simulink model "AllinOne_2014a"  (R2014a)
settings: Solver=ode3  SolverMode=SingleTasking  StartTime=0.0  StopTime=Inf  RelTol=1e-3
StopFcn:
  | CoffeeMachineIOSupport('closefig');
settings Model: DataDictionary=Struct.sldd  NumberOfSteps=100  ParamWorkspaceSource=ReferencedWorkspace  Creator=89YY  LastModifiedBy=zhiping
settings OptimizationCC: InlineParams=on  UseFloatMulNetSlope=on  InlineInvariantSignals=on  PassReuseOutputArgsAs=Individual arguments  ZeroExternalMemoryAtStartup=off  ZeroInternalMemoryAtStartup=off  NoFixptDivByZeroProtection=on  EfficientFloat2IntCast=on  OptimizeModelRefInitCode=on  LifeSpan=1
settings DebuggingCC: SaveWithParameterizedLinksMsg=none  UnderspecifiedInitializationDetection=Classic  SolverPrmCheckMsg=none  FrameProcessingCompatibilityMsg=error
settings HardwareCC: ProdBitPerPointer=64  ProdLargestAtomicFloat=Float  ProdIntDivRoundTo=Zero  ProdEndianess=LittleEndian  ProdHWDeviceType=Specified  TargetBitPerPointer=64  TargetLongLongMode=on  TargetIntDivRoundTo=Zero  TargetEndianess=LittleEndian  TargetWordSize=64  TargetHWDeviceType=MATLAB Host  ProdEqTarget=off
settings RTWCC: SystemTargetFile=ert.tlc  TemplateMakefile=ert_default_tmf  Description=Embedded Coder  GenerateReport=on  IncludeHyperlinkInReport=on  LaunchReport=on  GenerateTraceInfo=on  GenerateTraceReport=on  GenerateTraceReportSl=on  GenerateTraceReportSf=on  GenerateTraceReportEml=on  GenerateCodeMetricsReport=on
settings CodeAppCC: ForceParamTrailComments=on  IgnoreCustomStorageClasses=off  SimulinkDataObjDesc=on  CustomSymbolStrGlobalVar=rt$N$M  CustomSymbolStrType=$N$M  CustomSymbolStrFcn=$N$M$F  CustomSymbolStrMacro=$N$M  InsertBlockDesc=on
settings ERTTargetCC: ParMdlRefBuildCompliant=on  CompOptLevelCompliant=on  ConcurrentExecutionCompliant=on  IncludeMdlTerminateFcn=off  CombineSignalStateStructs=on  ERTFirstTimeCompliant=on  SupportNonFinite=off  SupportContinuousTime=on  ModelStepFunctionPrototypeControlCompliant=on  CPPClassGenCompliant=on  ERTCustomFileTemplate=example_file_process.tlc  ERTFilePackagingFormat=CompactWithDataFile

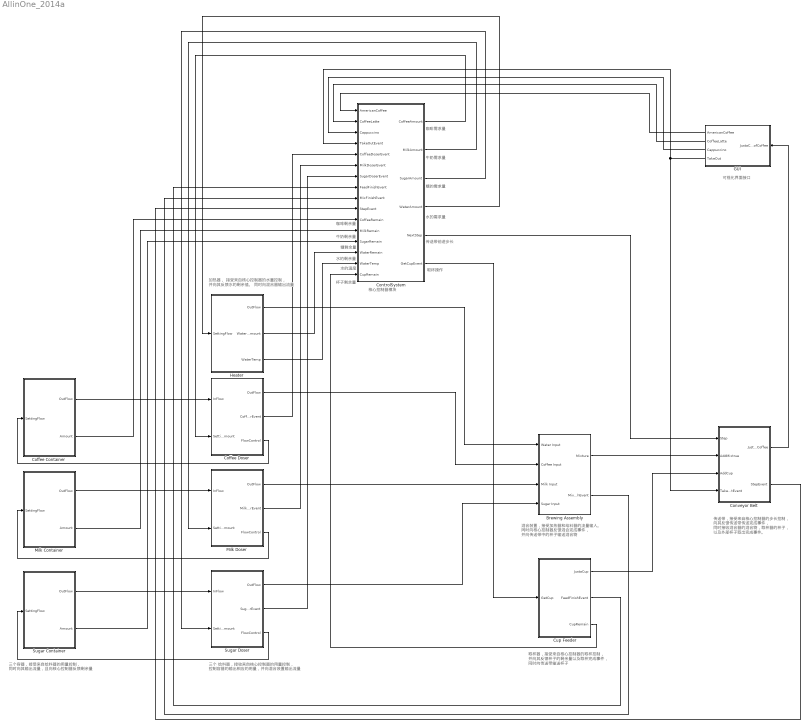
== system AllinOne_2014a ==
  note: 水的需求量
  note: 可视化界面接口
  note: 加热器， 接受来自核心控制器的水量控制，
      | 并向其反馈水的剩余值。
      | 同时向混合器输出流量
  note: 传送带，接受来自核心控制器的步长控制，
      | 向其反馈传送带传送完成事件，
      | 同时接收混合器的混合物，取杯器的杯子，
      | 以及外部杯子取出完成事件。
  note: 混合装置，接受加热器和给料器的流量输入。
      | 同时向核心控制器反馈混合完成事件，
      | 并向传送带中的杯子输送混合物
  note: 取杯器，接受来自核心控制器的取杯控制，
      | 并向其反馈杯子的剩余量以及取杯完成事件，
      | 同时向传送带输送杯子
  note: 三个 给料器，接收来自核心控制器的用量控制，
      | 控制容器的输出相应的用量，并向混合装置输出流量
  note: 三个容器，接受来自给料器的用量控制，
      | 同时向其输出流量，且向核心控制器反馈剩余量
  note: 取杯操作
  note: 传送带前进步长
  note: 糖的需求量
  note: 牛奶需求量
  note: 咖啡需求量
  note: 杯子剩余量
  note: 水的温度
  note: 水的剩余量
  note: 糖剩余量
  note: 牛奶剩余量
  note: 咖啡剩余量
  note: 核心控制器模块
  Brewing Assembly : Subsystem
  Coffee Container : Subsystem
  Coffee Doser : Subsystem
  ControlSystem : Subsystem
  Conveyor Belt : Subsystem
  Cup Feeder : Subsystem
  GUI : Subsystem
  Heater : Subsystem
  Milk Container : Subsystem
  Milk Doser : Subsystem
  Sugar Container : Subsystem
  Sugar Doser : Subsystem
  wires:
  Milk Container/1(OutFlow) -> Milk Doser/1(InFlow)
  Milk Doser/3(FlowControl) -> Milk Container/1(SettingFlow)
  Coffee Container/1(OutFlow) -> Coffee Doser/1(InFlow)
  Coffee Doser/3(FlowControl) -> Coffee Container/1(SettingFlow)
  Sugar Container/1(OutFlow) -> Sugar Doser/1(InFlow)
  Sugar Doser/3(FlowControl) -> Sugar Container/1(SettingFlow)
  Coffee Doser/1(OutFlow) -> Brewing Assembly/2(Coffee Input)
  Milk Doser/1(OutFlow) -> Brewing Assembly/3(Milk Input)
  Sugar Doser/1(OutFlow) -> Brewing Assembly/4(Sugar Input)
  Brewing Assembly/1(Mixture) -> Conveyor Belt/2(AddMixtrue)
  Cup Feeder/1(JustaCup) -> Conveyor Belt/3(AddCup)
  Heater/1(OutFlow) -> Brewing Assembly/1(Water Input)
  GUI/4(TakeOut) -> Conveyor Belt/4(TakeOutEvent), ControlSystem/4(TakeOutEvent)
  Conveyor Belt/1(JustaCupofCoffee) -> GUI/1(JustaCupofCoffee)
  GUI/3(Cappuccino) -> ControlSystem/3(Cappuccino)
  GUI/2(CoffeeLatte) -> ControlSystem/2(CoffeeLatte)
  GUI/1(AmericanCoffee) -> ControlSystem/1(AmericanCoffee)
  Coffee Doser/2(CoffeeDoserEvent) -> ControlSystem/5(CoffeeDoserEvent)
  Milk Doser/2(MilkDoserEvent) -> ControlSystem/6(MilkDoserEvent)
  Sugar Doser/2(SugarDoserEvent) -> ControlSystem/7(SugarDoserEvent)
  Coffee Container/2(Amount) -> ControlSystem/11(CoffeeRemain)
  Milk Container/2(Amount) -> ControlSystem/12(MilkRemain)
  Sugar Container/2(Amount) -> ControlSystem/13(SugarRemain)
  Heater/2(WaterAmount) -> ControlSystem/14(WaterRemain)
  Heater/3(WaterTemp) -> ControlSystem/15(WaterTemp)
  Cup Feeder/3(CupRemain) -> ControlSystem/16(CupRemain)
  Brewing Assembly/2(MixFinishEvent) -> ControlSystem/9(MixFinishEvent)
  Cup Feeder/2(FeedFinishEvent) -> ControlSystem/8(FeedFinishEvent)
  Conveyor Belt/2(StepEvent) -> ControlSystem/10(StepEvent)
  ControlSystem/1(CoffeeAmount) -> Coffee Doser/2(SettingAmount)
  ControlSystem/2(MilkAmount) -> Milk Doser/2(SettingAmount)
  ControlSystem/3(SugarAmount) -> Sugar Doser/2(SettingAmount)
  ControlSystem/6(GetCupEvent) -> Cup Feeder/1(GetCup)
  ControlSystem/5(NextStep) -> Conveyor Belt/1(Step)
  ControlSystem/4(WaterAmount) -> Heater/1(SettingFlow)

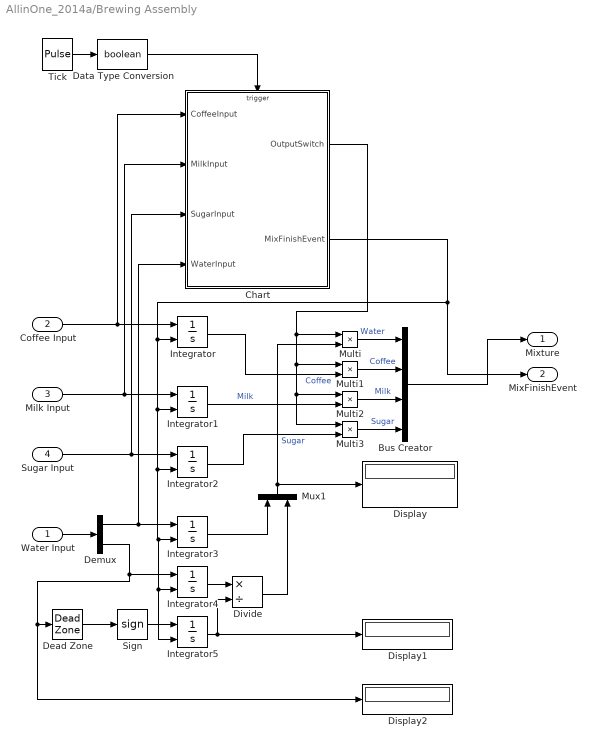
== system AllinOne_2014a/Brewing Assembly ==
  Water Input : Inport
  Coffee Input : Inport  Port=2
  Milk Input : Inport  Port=3
  Sugar Input : Inport  Port=4
  Bus Creator : BusCreator  Inputs=4  OutDataTypeStr=Bus: Mixtrue
  Chart : Stateflow chart  TreatAsAtomicUnit=on
      settings: PermitHierarchicalResolution=ParametersOnly
  Data Type Conversion : DataTypeConversion  OutDataTypeStr=boolean
  Dead Zone : DeadZone  LowerValue=-1e-5  UpperValue=1e-5  SaturateOnIntegerOverflow=on
  Demux : Demux  Outputs=2
  Display : Display
  Display1 : Display
  Display2 : Display
  Divide : Product  Inputs=*/
  Integrator{,1..5} (6 alike) : Integrator  ExternalReset=rising
  Multi{,1..3} (4 alike) : Product  Inputs=**
  Mux1 : Mux  Inputs=2
  Sign : Signum
  Tick : DiscretePulseGenerator  PulseType=Time based  Period=0.01  PulseWidth=50
  Mixture : Outport  OutDataTypeStr=Bus: Mixtrue
  MixFinishEvent : Outport  Port=2
  wires:
  Tick/1 -> Data Type Conversion/1
  Data Type Conversion/1 -> Chart/Trigger
  Sugar Input/1 -> Integrator2/1, Chart/3(SugarInput)
  Demux/1 -> Chart/4(WaterInput), Integrator3/1
  Milk Input/1 -> Integrator1/1, Chart/2(MilkInput)
  Coffee Input/1 -> Integrator/1, Chart/1(CoffeeInput)
  Chart/2(MixFinishEvent) -> MixFinishEvent/1, Integrator5/2, Integrator4/2, Integrator3/2, Integrator2/2, Integrator1/2, Integrator/2
  Multi1/1 -> Bus Creator/2  "Coffee"
  Mux1/1 -> Multi/2, Display/1
  Multi2/1 -> Bus Creator/3  "Milk"
  Multi3/1 -> Bus Creator/4  "Sugar"
  Bus Creator/1 -> Mixture/1
  Chart/1(OutputSwitch) -> Multi3/1, Multi2/1, Multi1/1, Multi/1
  Water Input/1 -> Demux/1
  Integrator3/1 -> Mux1/1
  Sign/1 -> Integrator5/1
  Demux/2 -> Display2/1, Dead Zone/1, Integrator4/1
  Integrator4/1 -> Divide/1
  Integrator5/1 -> Display1/1, Divide/2
  Divide/1 -> Mux1/2
  Multi/1 -> Bus Creator/1  "Water"
  Integrator/1 -> Multi1/2  "Coffee"
  Integrator1/1 -> Multi2/2  "Milk"
  Integrator2/1 -> Multi3/2  "Sugar"
  Dead Zone/1 -> Sign/1

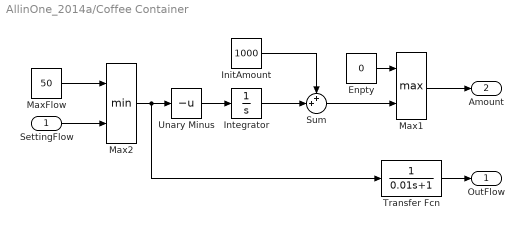
== system AllinOne_2014a/Coffee Container ==
  SettingFlow : Inport
  Enpty : Constant  Value=0
  InitAmount : Constant  Value=1000
  Integrator : Integrator
  Max1 : MinMax  Function=max  Inputs=2
  Max2 : MinMax  Inputs=2  OutMin=[0]
  MaxFlow : Constant  Value=50
  Sum : Sum  Inputs=++|
  Transfer Fcn : TransferFcn  Denominator=[0.01 1]
  Unary Minus : UnaryMinus
  OutFlow : Outport
  Amount : Outport  Port=2
  wires:
  Unary Minus/1 -> Integrator/1
  Integrator/1 -> Sum/2
  SettingFlow/1 -> Max2/2
  InitAmount/1 -> Sum/1
  Max2/1 -> Transfer Fcn/1, Unary Minus/1
  MaxFlow/1 -> Max2/1
  Max1/1 -> Amount/1
  Sum/1 -> Max1/2
  Enpty/1 -> Max1/1
  Transfer Fcn/1 -> OutFlow/1

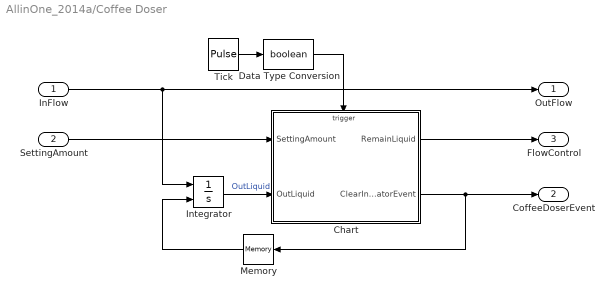
== system AllinOne_2014a/Coffee Doser ==
  InFlow : Inport
  SettingAmount : Inport  Port=2
  Chart : Stateflow chart  RequirementInfo={} %GIDa_ffed56c2_cd34_4288_8248_c4489554cc95  TreatAsAtomicUnit=on
      settings: PermitHierarchicalResolution=ParametersOnly
  Data Type Conversion : DataTypeConversion  OutDataTypeStr=boolean
  Integrator : Integrator  ExternalReset=rising
  Memory : Memory
  Tick : DiscretePulseGenerator  PulseType=Time based  Period=0.01  PulseWidth=50
  OutFlow : Outport
  CoffeeDoserEvent : Outport  Port=2
  FlowControl : Outport  Port=3
  wires:
  SettingAmount/1 -> Chart/1(SettingAmount)
  Chart/1(RemainLiquid) -> FlowControl/1
  InFlow/1 -> OutFlow/1, Integrator/1
  Chart/2(ClearIntegratorEvent) -> Memory/1, CoffeeDoserEvent/1
  Integrator/1 -> Chart/2(OutLiquid)  "OutLiquid"
  Tick/1 -> Data Type Conversion/1
  Data Type Conversion/1 -> Chart/Trigger
  Memory/1 -> Integrator/2

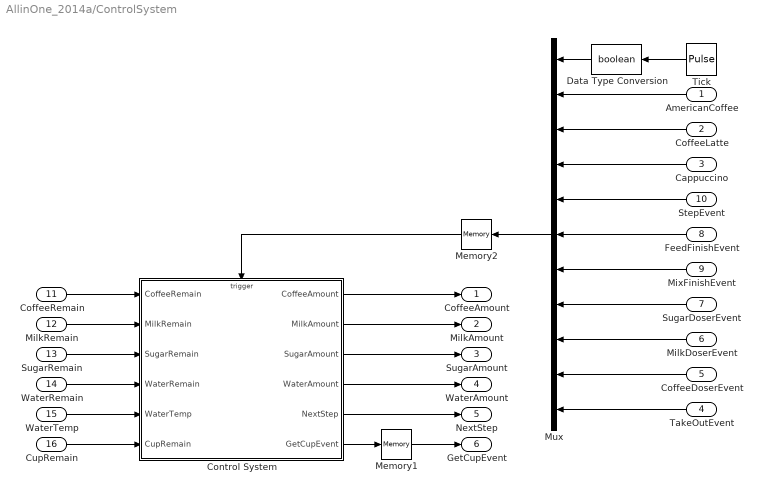
== system AllinOne_2014a/ControlSystem ==
  AmericanCoffee : Inport
  CoffeeLatte : Inport  Port=2
  Cappuccino : Inport  Port=3
  TakeOutEvent : Inport  Port=4
  CoffeeDoserEvent : Inport  Port=5
  MilkDoserEvent : Inport  Port=6
  SugarDoserEvent : Inport  Port=7
  FeedFinishEvent : Inport  Port=8
  MixFinishEvent : Inport  Port=9
  StepEvent : Inport  Port=10
  CoffeeRemain : Inport  Port=11
  MilkRemain : Inport  Port=12
  SugarRemain : Inport  Port=13
  WaterRemain : Inport  Port=14
  WaterTemp : Inport  Port=15
  CupRemain : Inport  Port=16
  Control System : Stateflow chart  TreatAsAtomicUnit=on
      settings: PermitHierarchicalResolution=ParametersOnly
  Data Type Conversion : DataTypeConversion  OutDataTypeStr=boolean
  Memory1 : Memory
  Memory2 : Memory
  Mux : Mux  Inputs=11
  Tick : DiscretePulseGenerator  PulseType=Time based  Period=0.01  PulseWidth=50
  CoffeeAmount : Outport
  MilkAmount : Outport  Port=2
  SugarAmount : Outport  Port=3
  WaterAmount : Outport  Port=4
  NextStep : Outport  Port=5
  GetCupEvent : Outport  Port=6
  wires:
  TakeOutEvent/1 -> Mux/11
  CoffeeLatte/1 -> Mux/3
  Cappuccino/1 -> Mux/4
  AmericanCoffee/1 -> Mux/2
  Control System/3(SugarAmount) -> SugarAmount/1
  FeedFinishEvent/1 -> Mux/6
  MilkRemain/1 -> Control System/2(MilkRemain)
  Control System/6(GetCupEvent) -> Memory1/1
  Control System/2(MilkAmount) -> MilkAmount/1
  MixFinishEvent/1 -> Mux/7
  SugarRemain/1 -> Control System/3(SugarRemain)
  CoffeeRemain/1 -> Control System/1(CoffeeRemain)
  Control System/1(CoffeeAmount) -> CoffeeAmount/1
  Control System/4(WaterAmount) -> WaterAmount/1
  Tick/1 -> Data Type Conversion/1
  WaterTemp/1 -> Control System/5(WaterTemp)
  StepEvent/1 -> Mux/5
  SugarDoserEvent/1 -> Mux/8
  MilkDoserEvent/1 -> Mux/9
  CoffeeDoserEvent/1 -> Mux/10
  Control System/5(NextStep) -> NextStep/1
  WaterRemain/1 -> Control System/4(WaterRemain)
  CupRemain/1 -> Control System/6(CupRemain)
  Data Type Conversion/1 -> Mux/1
  Memory1/1 -> GetCupEvent/1
  Mux/1 -> Memory2/1
  Memory2/1 -> Control System/Trigger

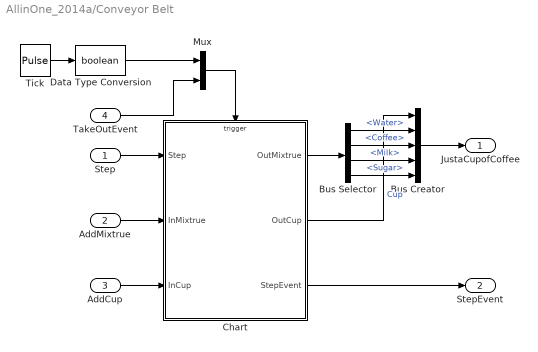
== system AllinOne_2014a/Conveyor Belt ==
  Step : Inport
  AddMixtrue : Inport  Port=2
  AddCup : Inport  Port=3
  TakeOutEvent : Inport  Port=4
  Bus Creator : BusCreator  Inputs=5
  Bus Selector : BusSelector  OutputSignals=Water,Coffee,Milk,Sugar
  Chart : Stateflow chart  TreatAsAtomicUnit=on
      settings: PermitHierarchicalResolution=ParametersOnly
  Data Type Conversion : DataTypeConversion  OutDataTypeStr=boolean
  Mux : Mux  Inputs=2
  Tick : DiscretePulseGenerator  PulseType=Time based  Period=0.01  PulseWidth=50
  JustaCupofCoffee : Outport  OutDataTypeStr=Bus: aCupofCoffee
  StepEvent : Outport  Port=2
  wires:
  Tick/1 -> Data Type Conversion/1
  Data Type Conversion/1 -> Mux/1
  Chart/3(StepEvent) -> StepEvent/1
  AddCup/1 -> Chart/3(InCup)
  AddMixtrue/1 -> Chart/2(InMixtrue)
  Step/1 -> Chart/1(Step)
  Chart/1(OutMixtrue) -> Bus Selector/1
  Bus Selector/1 -> Bus Creator/2  "<Water>"
  Bus Selector/2 -> Bus Creator/3  "<Coffee>"
  Bus Selector/3 -> Bus Creator/4  "<Milk>"
  Bus Selector/4 -> Bus Creator/5  "<Sugar>"
  Chart/2(OutCup) -> Bus Creator/1  "Cup"
  Bus Creator/1 -> JustaCupofCoffee/1
  Mux/1 -> Chart/Trigger
  TakeOutEvent/1 -> Mux/2

== system AllinOne_2014a/Cup Feeder ==
  GetCup : Inport
  Chart : Stateflow chart  TreatAsAtomicUnit=on
      settings: PermitHierarchicalResolution=ParametersOnly
  Data Type Conversion : DataTypeConversion  OutDataTypeStr=boolean
  Mux : Mux  Inputs=2
  Tick : DiscretePulseGenerator  PulseType=Time based  Period=0.01  PulseWidth=50
  JustaCup : Outport
  FeedFinishEvent : Outport  Port=2
  CupRemain : Outport  Port=3
  wires:
  Chart/1(JustaCup) -> JustaCup/1
  Chart/2(CupRemain) -> CupRemain/1
  Chart/3(FeedFinishEvent) -> FeedFinishEvent/1
  GetCup/1 -> Mux/2
  Tick/1 -> Data Type Conversion/1
  Mux/1 -> Chart/Trigger
  Data Type Conversion/1 -> Mux/1

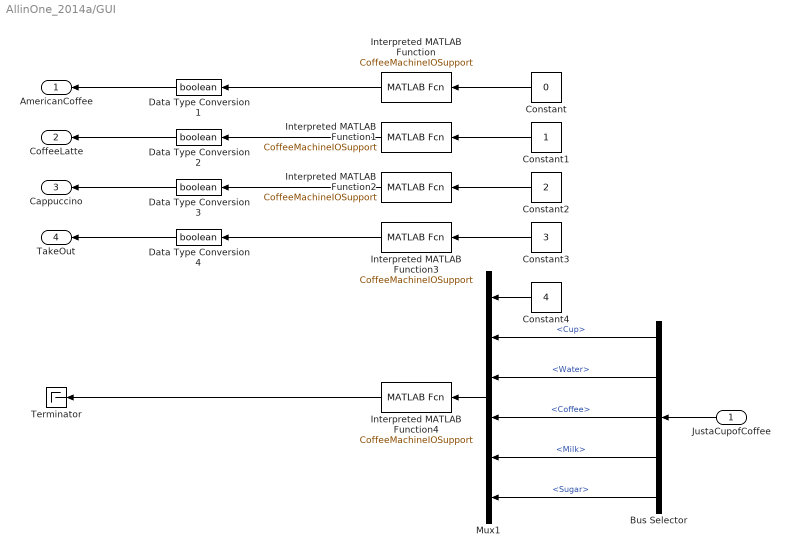
== system AllinOne_2014a/GUI ==
  JustaCupofCoffee : Inport
  Bus Selector : BusSelector  OutputSignals=Cup,Water,Coffee,Milk,Sugar
  Constant : Constant  Value=0
  Constant1 : Constant
  Constant2 : Constant  Value=2
  Constant3 : Constant  Value=3
  Constant4 : Constant  Value=4
  Data Type Conversion{1..4} (4 alike) : DataTypeConversion  OutDataTypeStr=boolean
  Interpreted MATLAB Function{,1..4} (5 alike) : MATLABFcn  MATLABFcn=CoffeeMachineIOSupport
  Mux1 : Mux  Inputs=6
  Terminator : Terminator
  AmericanCoffee : Outport
  CoffeeLatte : Outport  Port=2
  Cappuccino : Outport  Port=3
  TakeOut : Outport  Port=4
  wires:
  JustaCupofCoffee/1 -> Bus Selector/1
  Interpreted MATLAB Function3/1 -> Data Type Conversion4/1
  Interpreted MATLAB Function2/1 -> Data Type Conversion3/1
  Mux1/1 -> Interpreted MATLAB Function4/1
  Bus Selector/1 -> Mux1/2  "<Cup>"
  Bus Selector/3 -> Mux1/4  "<Coffee>"
  Bus Selector/4 -> Mux1/5  "<Milk>"
  Bus Selector/5 -> Mux1/6  "<Sugar>"
  Constant/1 -> Interpreted MATLAB Function/1
  Constant1/1 -> Interpreted MATLAB Function1/1
  Interpreted MATLAB Function/1 -> Data Type Conversion1/1
  Bus Selector/2 -> Mux1/3  "<Water>"
  Interpreted MATLAB Function1/1 -> Data Type Conversion2/1
  Constant4/1 -> Mux1/1
  Constant2/1 -> Interpreted MATLAB Function2/1
  Constant3/1 -> Interpreted MATLAB Function3/1
  Interpreted MATLAB Function4/1 -> Terminator/1
  Data Type Conversion2/1 -> CoffeeLatte/1
  Data Type Conversion1/1 -> AmericanCoffee/1
  Data Type Conversion3/1 -> Cappuccino/1
  Data Type Conversion4/1 -> TakeOut/1

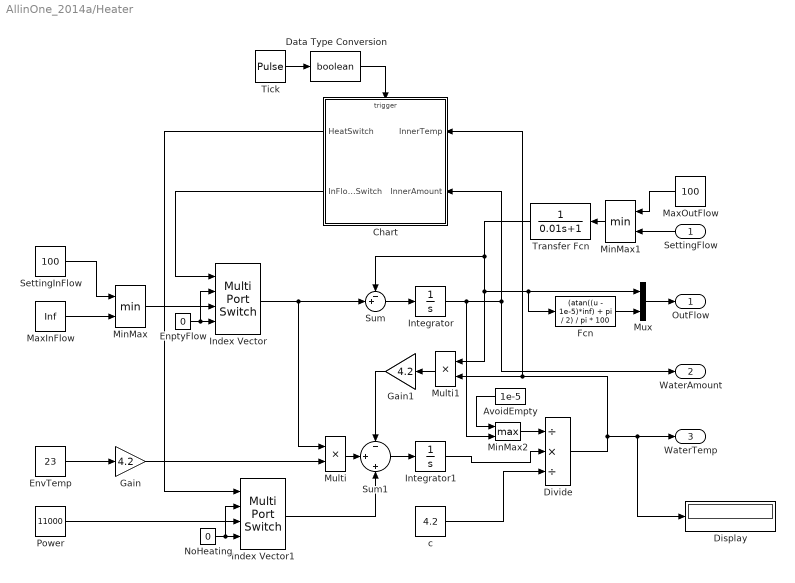
== system AllinOne_2014a/Heater ==
  SettingFlow : Inport
  AvoidEmpty : Constant  Value=1e-5
  Chart : Stateflow chart  TreatAsAtomicUnit=on
      settings: PermitHierarchicalResolution=ParametersOnly
  Data Type Conversion : DataTypeConversion  OutDataTypeStr=boolean
  Display : Display
  Divide : Product  Inputs=/*/
  EnptyFlow : Constant  Value=0
  EnvTemp : Constant  Value=23
  Fcn : Fcn  Expr=(atan((u - 1e-5)*inf) + pi / 2) / pi * 100
  Gain : Gain  Gain=4.2
  Gain1 : Gain  Gain=4.2
  Index Vector : MultiPortSwitch  DataPortOrder=Zero-based contiguous  Inputs=2  DataPortForDefault=Additional data port  DiagnosticForDefault=None  zeroidx=on
  Index Vector1 : MultiPortSwitch  DataPortOrder=Zero-based contiguous  Inputs=2  DataPortForDefault=Additional data port  DiagnosticForDefault=None  zeroidx=on
  Integrator : Integrator
  Integrator1 : Integrator
  MaxInFlow : Constant  Value=Inf
  MaxOutFlow : Constant  Value=100
  MinMax : MinMax  Inputs=2
  MinMax1 : MinMax  Inputs=2
  MinMax2 : MinMax  Function=max  Inputs=2
  Multi : Product  Inputs=**
  Multi1 : Product  Inputs=**
  Mux : Mux  Inputs=2
  NoHeating : Constant  Value=0
  Power : Constant  Value=11000
  SettingInFlow : Constant  Value=100
  Sum : Sum  Inputs=-+|
  Sum1 : Sum  Inputs=-|+|+
  Tick : DiscretePulseGenerator  PulseType=Time based  Period=0.01  PulseWidth=50
  Transfer Fcn : TransferFcn  Denominator=[0.01 1]
  c : Constant  Value=4.2
  OutFlow : Outport
  WaterAmount : Outport  Port=2
  WaterTemp : Outport  Port=3
  wires:
  MaxInFlow/1 -> MinMax/2
  SettingInFlow/1 -> MinMax/1
  Sum/1 -> Integrator/1
  Sum1/1 -> Integrator1/1
  EnvTemp/1 -> Gain/1
  Integrator/1 -> MinMax2/2, WaterAmount/1, Chart/2(InnerAmount)
  Integrator1/1 -> Divide/2
  c/1 -> Divide/3
  Gain/1 -> Multi/2
  Multi/1 -> Sum1/2
  Index Vector/1 -> Multi/1, Sum/2
  EnptyFlow/1 -> Index Vector/2, Index Vector/4
  MinMax/1 -> Index Vector/3
  Chart/2(InFlowSwitch) -> Index Vector/1
  NoHeating/1 -> Index Vector1/2, Index Vector1/4
  Chart/1(HeatSwitch) -> Index Vector1/1
  Index Vector1/1 -> Sum1/3
  Power/1 -> Index Vector1/3
  MaxOutFlow/1 -> MinMax1/1
  SettingFlow/1 -> MinMax1/2
  MinMax1/1 -> Transfer Fcn/1
  Mux/1 -> OutFlow/1
  Transfer Fcn/1 -> Fcn/1, Mux/1, Multi1/1, Sum/1
  Tick/1 -> Data Type Conversion/1
  Data Type Conversion/1 -> Chart/Trigger
  Multi1/1 -> Gain1/1
  Gain1/1 -> Sum1/1
  MinMax2/1 -> Divide/1
  AvoidEmpty/1 -> MinMax2/1
  Divide/1 -> Multi1/2, Chart/1(InnerTemp), Display/1, WaterTemp/1
  Fcn/1 -> Mux/2

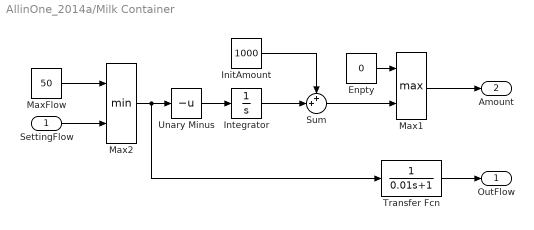
== system AllinOne_2014a/Milk Container ==
  SettingFlow : Inport
  Enpty : Constant  Value=0
  InitAmount : Constant  Value=1000
  Integrator : Integrator
  Max1 : MinMax  Function=max  Inputs=2
  Max2 : MinMax  Inputs=2  OutMin=[0]
  MaxFlow : Constant  Value=50
  Sum : Sum  Inputs=++|
  Transfer Fcn : TransferFcn  Denominator=[0.01 1]
  Unary Minus : UnaryMinus
  OutFlow : Outport
  Amount : Outport  Port=2
  wires:
  Unary Minus/1 -> Integrator/1
  Integrator/1 -> Sum/2
  SettingFlow/1 -> Max2/2
  InitAmount/1 -> Sum/1
  Max2/1 -> Transfer Fcn/1, Unary Minus/1
  MaxFlow/1 -> Max2/1
  Max1/1 -> Amount/1
  Sum/1 -> Max1/2
  Enpty/1 -> Max1/1
  Transfer Fcn/1 -> OutFlow/1

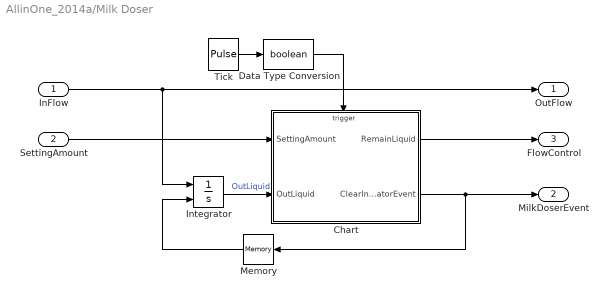
== system AllinOne_2014a/Milk Doser ==
  InFlow : Inport
  SettingAmount : Inport  Port=2
  Chart : Stateflow chart  RequirementInfo={} %GIDa_551bb34e_10e7_4a73_950c_ffc9537d9666  TreatAsAtomicUnit=on
      settings: PermitHierarchicalResolution=ParametersOnly
  Data Type Conversion : DataTypeConversion  OutDataTypeStr=boolean
  Integrator : Integrator  ExternalReset=rising
  Memory : Memory
  Tick : DiscretePulseGenerator  PulseType=Time based  Period=0.01  PulseWidth=50
  OutFlow : Outport
  MilkDoserEvent : Outport  Port=2
  FlowControl : Outport  Port=3
  wires:
  SettingAmount/1 -> Chart/1(SettingAmount)
  Chart/1(RemainLiquid) -> FlowControl/1
  InFlow/1 -> OutFlow/1, Integrator/1
  Chart/2(ClearIntegratorEvent) -> Memory/1, MilkDoserEvent/1
  Integrator/1 -> Chart/2(OutLiquid)  "OutLiquid"
  Tick/1 -> Data Type Conversion/1
  Data Type Conversion/1 -> Chart/Trigger
  Memory/1 -> Integrator/2

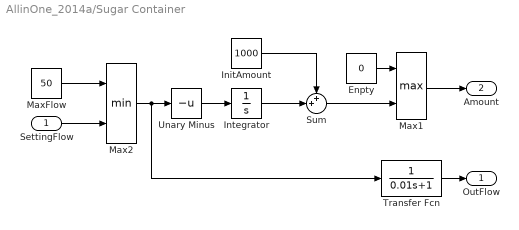
== system AllinOne_2014a/Sugar Container ==
  SettingFlow : Inport
  Enpty : Constant  Value=0
  InitAmount : Constant  Value=1000
  Integrator : Integrator
  Max1 : MinMax  Function=max  Inputs=2
  Max2 : MinMax  Inputs=2  OutMin=[0]
  MaxFlow : Constant  Value=50
  Sum : Sum  Inputs=++|
  Transfer Fcn : TransferFcn  Denominator=[0.01 1]
  Unary Minus : UnaryMinus
  OutFlow : Outport
  Amount : Outport  Port=2
  wires:
  Unary Minus/1 -> Integrator/1
  Integrator/1 -> Sum/2
  SettingFlow/1 -> Max2/2
  InitAmount/1 -> Sum/1
  Max2/1 -> Transfer Fcn/1, Unary Minus/1
  MaxFlow/1 -> Max2/1
  Max1/1 -> Amount/1
  Sum/1 -> Max1/2
  Enpty/1 -> Max1/1
  Transfer Fcn/1 -> OutFlow/1

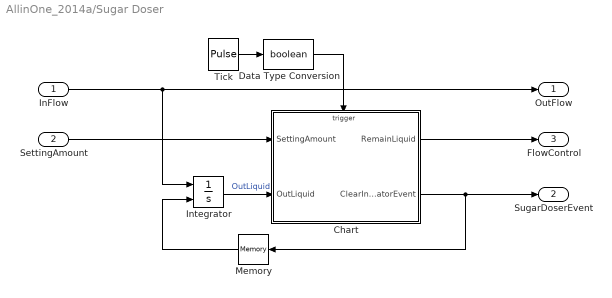
== system AllinOne_2014a/Sugar Doser ==
  InFlow : Inport
  SettingAmount : Inport  Port=2
  Chart : Stateflow chart  RequirementInfo={} %GIDa_3f65ce12_bb97_4ef2_8d1d_79df95e5fb82  TreatAsAtomicUnit=on
      settings: PermitHierarchicalResolution=ParametersOnly
  Data Type Conversion : DataTypeConversion  OutDataTypeStr=boolean
  Integrator : Integrator  ExternalReset=rising
  Memory : Memory
  Tick : DiscretePulseGenerator  PulseType=Time based  Period=0.01  PulseWidth=50
  OutFlow : Outport
  SugarDoserEvent : Outport  Port=2
  FlowControl : Outport  Port=3
  wires:
  SettingAmount/1 -> Chart/1(SettingAmount)
  Chart/1(RemainLiquid) -> FlowControl/1
  InFlow/1 -> OutFlow/1, Integrator/1
  Chart/2(ClearIntegratorEvent) -> Memory/1, SugarDoserEvent/1
  Integrator/1 -> Chart/2(OutLiquid)  "OutLiquid"
  Tick/1 -> Data Type Conversion/1
  Data Type Conversion/1 -> Chart/Trigger
  Memory/1 -> Integrator/2

== stateflow chart AllinOne_2014a/Conveyor Belt/Chart ==
  settings: executeAtInitialization=1  initializeOutput=1
  state MixtrueMonitor [parallel]
    settings: executionOrder=2
    state Waiting
    state Adding
      en:
      LocalMixtrue = InMixtrue;
    MixtrueMonitor.Waiting -> MixtrueMonitor.Adding : [InMixtrue.Coffee > eps && ...
        | abs(CupLocation - 50) < 5]
    (default) -> MixtrueMonitor.Waiting
    MixtrueMonitor.Adding -> MixtrueMonitor.Waiting : [InMixtrue.Coffee > eps]
  state CupMonitor [parallel]
    settings: executionOrder=3
    state Waiting
    state Adding
      en:
      CupLocation = 0;
    CupMonitor.Waiting -> CupMonitor.Adding : [InCup > eps && ...
        | CupLocation < 0]
    (default) -> CupMonitor.Waiting
    CupMonitor.Adding -> CupMonitor.Waiting : [InCup > eps]
  state CupTransmit [parallel]
    settings: executionOrder=1
    state Start
      en:CupLocation = -1;
    state Running
    state Output
      en:
      OutMixtrue = LocalMixtrue;
      OutCup = 1;
      ex:
      OutMixtrue.Water = [0,0]';
      OutMixtrue.Coffee = 0;
      OutMixtrue.Milk = 0;
      OutMixtrue.Sugar = 0;
      OutCup = 0;
    state Prepare
    state Finished
    state Stepping
      en:
      CupLocation = CupLocation + Step;
      StepEvent;
      ex:
      StepEvent;
    Output -> Start : TakeOutEvent
    Start -> Running : [CupLocation >= 0]
    (default) -> Start
    Running -> Output [order 1] : [CupLocation >= 100]
    Finished -> Running : [Step < eps]
    Running -> Prepare [order 2] : [Step > eps && CupLocation >= 0]
    Prepare -> Stepping : [after(Step, Tick)]
    Stepping -> Finished : after(10, Tick)
  data: Step input; CupLocation local; InMixtrue input Bus: Mixtrue; OutMixtrue output Bus: Mixtrue; InCup input; OutCup output; LocalMixtrue local Bus: Mixtrue
  events: Tick input RISING_EDGE_EVENT; StepEvent output EITHER_EDGE_EVENT; TakeOutEvent input RISING_EDGE_EVENT

== stateflow chart AllinOne_2014a/Milk Doser/Chart ==
  settings: sampleTime=TIMER  executeAtInitialization=1
  state Ready
  state Finish
  state Transmiting
    entry: TargetAmount = SettingAmount; RemainLiquid = TargetAmount / 3;
    exit: RemainLiquid = 0;
  (default) -> Ready
  Finish -> Ready : [after(5, Tick) && SettingAmount==0]
      | {
      | 	send(ClearIntegratorEvent);
      | }
  Ready -> Transmiting : [SettingAmount > 0]
  Transmiting -> Finish : [TargetAmount - OutLiquid <= 0]
      | {
      | 	send(ClearIntegratorEvent);
      | }
  data: SettingAmount input; RemainLiquid output; OutLiquid input; TargetAmount local
  events: ClearIntegratorEvent output EITHER_EDGE_EVENT; Tick input RISING_EDGE_EVENT

== stateflow chart AllinOne_2014a/Sugar Doser/Chart ==
  settings: sampleTime=TIMER  executeAtInitialization=1
  state Ready
  state Finish
  state Transmiting
    entry: TargetAmount = SettingAmount; RemainLiquid = TargetAmount / 3;
    exit: RemainLiquid = 0;
  (default) -> Ready
  Finish -> Ready : [after(5, Tick) && SettingAmount==0]
      | {
      | 	send(ClearIntegratorEvent);
      | }
  Ready -> Transmiting : [SettingAmount > 0]
  Transmiting -> Finish : [TargetAmount - OutLiquid <= 0]
      | {
      | 	send(ClearIntegratorEvent);
      | }
  data: SettingAmount input; RemainLiquid output; OutLiquid input; TargetAmount local
  events: ClearIntegratorEvent output EITHER_EDGE_EVENT; Tick input RISING_EDGE_EVENT

== stateflow chart AllinOne_2014a/Coffee Doser/Chart ==
  settings: sampleTime=TIMER  executeAtInitialization=1
  state Ready
  state Finish
  state Transmiting
    entry: TargetAmount = SettingAmount; RemainLiquid = TargetAmount / 3;
    exit: RemainLiquid = 0;
  (default) -> Ready
  Finish -> Ready : [after(5, Tick) && SettingAmount==0]
      | {
      | 	send(ClearIntegratorEvent);
      | }
  Ready -> Transmiting : [SettingAmount > 0]
  Transmiting -> Finish : [TargetAmount - OutLiquid <= 0]
      | {
      | 	send(ClearIntegratorEvent);
      | }
  data: SettingAmount input; RemainLiquid output; OutLiquid input; TargetAmount local
  events: ClearIntegratorEvent output EITHER_EDGE_EVENT; Tick input RISING_EDGE_EVENT

== stateflow chart AllinOne_2014a/Cup Feeder/Chart ==
  settings: executeAtInitialization=1  initializeOutput=1
  state Ready
    du:
    CupRemain=[CupAmount>0;];
  state PutaCup
    entry:
    send(FeedFinishEvent);
    JustaCup = 1;
    CupAmount = CupAmount - 1;
    exit:
    JustaCup = 0;
    send(FeedFinishEvent);
  (default) -> Ready : {
      | 	CupAmount = 10;
      | 	JustaCup = 0;
      | }
  PutaCup -> Ready : after(5, Tick)
  Ready -> PutaCup : NeedCupEvent
  data: JustaCup output; CupRemain output; CupAmount local
  events: FeedFinishEvent output EITHER_EDGE_EVENT; Tick input RISING_EDGE_EVENT; NeedCupEvent input RISING_EDGE_EVENT

== stateflow chart AllinOne_2014a/Heater/Chart ==
  state InFlow [parallel]
    settings: executionOrder=2
    state GetInFlow
      en: InFlowSwitch = 1;
    state OFF
      en: InFlowSwitch = 0;
    GetInFlow -> InFlow.OFF : [InnerAmount>2000]
    (default) -> InFlow.OFF
    InFlow.OFF -> GetInFlow : [InnerAmount<1900]
  state Heater [parallel]
    settings: executionOrder=1
    state Heating
      en: HeatSwitch = 1;
    state OFF
      en: HeatSwitch = 0;
    Heating -> Heater.OFF : [InnerTemp>82]
    (default) -> Heater.OFF
    Heater.OFF -> Heating : [InnerTemp<78]
  data: InnerTemp input; InnerAmount input; HeatSwitch output; InFlowSwitch output
  events: Tick input RISING_EDGE_EVENT

== stateflow chart AllinOne_2014a/Brewing Assembly/Chart ==
  settings: executeAtInitialization=1  initializeOutput=1
  state WaterState [parallel]
    settings: executionOrder=1
    state Waiting
    state Adding
    state Finished
    (default) -> WaterState.Waiting
    WaterState.Finished -> WaterState.Waiting : LocalFinishEvent
    WaterState.Waiting -> WaterState.Adding : [WaterInput > 1e-5]
    WaterState.Adding -> WaterState.Finished : [WaterInput < 1e-5]
  state CoffeeState [parallel]
    settings: executionOrder=2
    state Waiting
    state Adding
    state Finished
    (default) -> CoffeeState.Waiting
    CoffeeState.Finished -> CoffeeState.Waiting : LocalFinishEvent
    CoffeeState.Waiting -> CoffeeState.Adding : [CoffeeInput > 1e-5]
    CoffeeState.Adding -> CoffeeState.Finished : [CoffeeInput < 1e-5]
  state MilkState [parallel]
    settings: executionOrder=3
    state Waiting
    state Adding
    state Finished
    (default) -> MilkState.Waiting
    MilkState.Finished -> MilkState.Waiting : LocalFinishEvent
    MilkState.Waiting -> MilkState.Adding : [MilkInput > 1e-5]
    MilkState.Adding -> MilkState.Finished : [MilkInput < 1e-5]
  state SugarState [parallel]
    settings: executionOrder=4
    state Waiting
    state Adding
    state Finished
    (default) -> SugarState.Waiting
    SugarState.Finished -> SugarState.Waiting : LocalFinishEvent
    SugarState.Waiting -> SugarState.Adding : [SugarInput > 1e-5]
    SugarState.Adding -> SugarState.Finished : [SugarInput < 1e-5]
  state Mix [parallel]
    settings: executionOrder=5
    state Waiting
    state Mixing
    state Output
      en:
      OutputSwitch = 1;
      ex:
      OutputSwitch = 0;
    state Finished
      en:
      MixFinishEvent;
      LocalFinishEvent;
    Mix.Waiting -> Mixing : [in(WaterState.Finished) && ...
        | in(CoffeeState.Finished) && ...
        | in(MilkState.Finished) && ...
        | in(SugarState.Finished)]
    Output -> Mix.Finished : after(5, Tick)
    Mixing -> Output : after(5, Tick)
    (default) -> Mix.Waiting : {OutputSwitch = 0;}
    Mix.Finished -> Mix.Waiting : [after(10,Tick) && ...
        | in(WaterState.Waiting) && ...
        | in(CoffeeState.Waiting) && ...
        | in(MilkState.Waiting) && ...
        | in(SugarState.Waiting)]/
        | {
        | 	MixFinishEvent;
        | 	LocalFinishEvent;
        | }
  data: CoffeeInput input; MilkInput input; SugarInput input; WaterInput input; OutputSwitch output
  events: Tick input RISING_EDGE_EVENT; MixFinishEvent output EITHER_EDGE_EVENT; LocalFinishEvent local FUNCTION_CALL_EVENT

== stateflow chart AllinOne_2014a/ControlSystem/Control System ==
  state Init
    en:
    CoffeeAmount = 0;
    MilkAmount = 0;
    SugarAmount = 0;
    WaterAmount = 0;
    NextStep = 0;
  note: 检查函数，核对材料剩余量是否满足咖啡的需求量，满足则输出1，不满足输出0
  note: 总体流程，
      | 控制器接收来自外部的咖啡选择信号
      | （初始）——>进入配方状态
      | （响应）——>判断咖啡机是否满足制造咖啡的要求
      | （满足）——>进入取杯器取杯工作状态
      | （完成）——>进入传送带前进状态
      | （完成）——>进入给料器工作状态
      | （完成）——>进入传送带前进状态
      | （完成）——>进入等待取杯状态
      | （完成）——>进入初始状态，等待下一杯咖啡
  state flg = checkall(waterRemain,waterRecipe,milkRemain,milkRecipe,sugarRemain,sugarRecipe,coffeeRemain,coffeeRecipe,cupRemain,waterTemp) [function]
    (default) -> (junction 200)
    (junction 200) -> (junction 310) [order 2]
    (junction 310) -> (junction 327) [order 2]
    (junction 327) -> (junction 337) [order 2]
    (junction 337) -> (junction 353) [order 2]
    (junction 353) -> (junction 406) [order 2]
    (junction 406) -> (junction 202) [order 2] : {flg=1;}
    (junction 200) -> (junction 201) [order 1] : [waterRemain<waterRecipe]
    (junction 310) -> (junction 312) [order 1] : [milkRemain<milkRecipe]
    (junction 327) -> (junction 326) [order 1] : [sugarRemain<sugarRecipe]
    (junction 337) -> (junction 335) [order 1] : [coffeeRemain<coffeeRecipe]
    (junction 353) -> (junction 355) [order 1] : [cupRemain<=0]
    (junction 406) -> (junction 409) [order 1] : [waterTemp<=80]
    (junction 326) -> (junction 202) : {flg=0;}
    (junction 201) -> (junction 202) : {flg=0;}
    (junction 409) -> (junction 202) : {flg=0;}
    (junction 312) -> (junction 202) : {flg=0;}
    (junction 355) -> (junction 202) : {flg=0;}
    (junction 335) -> (junction 202) : {flg=0;}
  note: 响应取杯完成事件，进入初始状态，可以进行另一杯咖啡的制作。
  state TakeOut
  note: 
  note: 响应来自外部三种咖啡的信号，
      | 根据信号的不同自动进入三种状态，生成相应的配方。
  note: 等待取杯状态
  note: 错误状态
  state error
  note: 响应传送带传送完成事件，杯子已经送到输出口，进入等待取杯状态
  note: 
  state prepare_AmerricanCoffee
    en:
    CoffeeRecipe= 10;
    MilkRecipe= 60;
    SugarRecipe= 10;
    WaterRecipe =30;
  state prepare_Cappuccino
    en:
    CoffeeRecipe =10;
    MilkRecipe = 70;
    SugarRecipe= 10;
    WaterRecipe= 20;
  state prepare_CoffeeLatte
    en:
    CoffeeRecipe = 10;
    MilkRecipe = 80;
    SugarRecipe = 10;
    WaterRecipe= 40;
  state BeltStep2
    en:NextStep=50;
    ex:
    NextStep=0;
  note: 传送带运输工作状态
  note: 配方状态
  note: 如果在机器工作任何状态中，
      | 等待时间超过一定值，
      | 则机器进入error状态，
      | 不响应外部信号
  note: 响应混合器的完成事件，此时杯子的饮料已经装填完毕，下一步，
      | 传送带带着杯子进入输出口，假设运动步长为50.
  state GetCup
    en:
    GetCupEvent;
    ex:
    GetCupEvent;
  state working_Coffee
    note: 四个并行状态，由于水的用量是由阀的通断控制的，通过控制阀开启的时间就可以控制相应的用量。
        | 而咖啡，牛奶和糖有相应的pid控制器进行控制，所以需要响应相应的完成事件。
    state WaterState [parallel]
      settings: executionOrder=1
      state Working
        en:
        WaterAmount = 1;
        ex:
        WaterAmount = 0;
      state Finished
      (default) -> working_Coffee.WaterState.Working
      working_Coffee.WaterState.Working -> working_Coffee.WaterState.Finished : after(WaterRecipe, Tick)
    state SugarDoserState [parallel]
      settings: executionOrder=2
      state Working
        en:
        SugarAmount=SugarRecipe;
        ex:SugarAmount=0;
      state Finished
      (default) -> working_Coffee.SugarDoserState.Working
      working_Coffee.SugarDoserState.Working -> working_Coffee.SugarDoserState.Finished : SugarDoserEvent
    state CoffeeDoserState [parallel]
      settings: executionOrder=3
      state Working
        en:
        CoffeeAmount=CoffeeRecipe;
        ex:CoffeeAmount=0;
      state Finished
      (default) -> working_Coffee.CoffeeDoserState.Working
      working_Coffee.CoffeeDoserState.Working -> working_Coffee.CoffeeDoserState.Finished : CoffeeDoserEvent
    state MilkDoserState [parallel]
      settings: executionOrder=4
      state Working
        en:
        MilkAmount=MilkRecipe;
        ex:MilkAmount=0;
      state Finished
      (default) -> working_Coffee.MilkDoserState.Working
      working_Coffee.MilkDoserState.Working -> working_Coffee.MilkDoserState.Finished : MilkDoserEvent
  note: doser和水箱向杯子添加材料状态。
  note: 取杯状态
  note: 如果检查函数通过，则进行下一步取杯操作，
      | 否则，回退初始状态。
  note: 响应取杯完成操作后，
      | 进入传送带运行过程，
      | 假设运动步长为50。
  state BeltStep1
    en:NextStep=50;
    ex:NextStep=0;
  note: 响应传送带运行完成事件，此时杯子就位，
      | Doser和水箱加热器开始工作。
  note: 传送带运输工作状态
  (default) -> Init
  Init -> prepare_AmerricanCoffee [order 3] : Cappuccino
  prepare_AmerricanCoffee -> Init [order 2]
  Init -> prepare_Cappuccino [order 2] : CoffeeLatte
  prepare_Cappuccino -> Init [order 2]
  prepare_CoffeeLatte -> Init [order 2]
  Init -> prepare_CoffeeLatte [order 1] : AmericanCoffee
  TakeOut -> Init : TakeOutEvent
  BeltStep2 -> TakeOut [order 1] : StepEvent
  (junction 676) -> error
  BeltStep2 -> (junction 676) [order 2] : after(10000,Tick)
  prepare_AmerricanCoffee -> GetCup [order 1] : [checkall(WaterRemain,WaterRecipe,...
      | MilkRemain,MilkRecipe,SugarRemain,...
      | SugarRecipe,CoffeeRemain,...
      | CoffeeRecipe,CupRemain,WaterTemp)]
  prepare_Cappuccino -> GetCup [order 1] : [checkall(WaterRemain,WaterRecipe,...
      | MilkRemain,MilkRecipe,SugarRemain,...
      | SugarRecipe,CoffeeRemain,...
      | CoffeeRecipe,CupRemain,WaterTemp)]
  prepare_CoffeeLatte -> GetCup [order 1] : [checkall(WaterRemain,WaterRecipe,...
      | MilkRemain,MilkRecipe,SugarRemain,...
      | SugarRecipe,CoffeeRemain,...
      | CoffeeRecipe,CupRemain,WaterTemp)]
  working_Coffee -> BeltStep2 [order 1] : MixFinishEvent
  GetCup -> (junction 676) [order 2] : after(10000,Tick)
  working_Coffee -> (junction 676) [order 2] : after(10000,Tick)
  BeltStep1 -> (junction 676) [order 2] : after(10000,Tick)
  BeltStep1 -> working_Coffee [order 1] : StepEvent
  GetCup -> BeltStep1 [order 1] : FeedFinishEvent
  data: waterRemain function_input double size=1; waterRecipe function_input double size=1; milkRemain function_input double size=1; milkRecipe function_input double size=1; sugarRemain function_input double size=1; sugarRecipe function_input double size=1; coffeeRemain function_input double size=1; coffeeRecipe function_input double size=1; cupRemain function_input double size=1; waterTemp function_input double size=1; flg function_output boolean; CoffeeRemain input; MilkRemain input; SugarRemain input; CoffeeAmount output; MilkAmount output; SugarAmount output; WaterAmount output; NextStep output; WaterRemain input; WaterTemp input; CupRemain input; CoffeeRecipe local double size=1; MilkRecipe local double size=1; SugarRecipe local double size=1; WaterRecipe local double size=1
  events: Tick input RISING_EDGE_EVENT; AmericanCoffee input RISING_EDGE_EVENT; CoffeeLatte input RISING_EDGE_EVENT; Cappuccino input RISING_EDGE_EVENT; StepEvent input RISING_EDGE_EVENT; FeedFinishEvent input RISING_EDGE_EVENT; MixFinishEvent input RISING_EDGE_EVENT; SugarDoserEvent input RISING_EDGE_EVENT; MilkDoserEvent input RISING_EDGE_EVENT; CoffeeDoserEvent input RISING_EDGE_EVENT; GetCupEvent output EITHER_EDGE_EVENT; TakeOutEvent input RISING_EDGE_EVENT
